simulink model "Current_torque_111"  (R2017b)
settings: Solver=ode45  StartTime=0.0  StopTime=3  MaxStep=1e-4  RelTol=1e-3  EnableMultiTasking=on
libraries: neural x38, fuzblock x6, simulink x1
(part 1 of 3)
settings Model: Creator=Tianfu Sun  LastModifiedBy=dachuan
settings DataIOCC: LimitDataPoints=on  SaveFormat=Array  SignalLoggingSaveFormat=ModelDataLogs
settings OptimizationCC: ExpressionDepthLimit=2147483647  LifeSpan=inf
settings DebuggingCC: UnderspecifiedInitializationDetection=Classic  MergeDetectMultiDrivingBlocksExec=none  SolverPrmCheckMsg=warning  FcnCallInpInsideContextMsg=warning  StateNameClashWarn=warning  StrictBusMsg=Warning  SFUnexpectedBacktrackingDiag=warning  SFNoUnconditionalDefaultTransitionDiag=warning  SFExecutionAtInitializationDiag=none
settings HardwareCC: ProdBitPerPointer=32  ProdBitPerSizeT=32  ProdBitPerPtrDiffT=32  ProdLargestAtomicFloat=None  ProdIntDivRoundTo=Undefined  ProdEndianess=Unspecified  ProdWordSize=32  ProdHWDeviceType=32-bit Generic
settings ModelReferenceCC: PropagateSignalLabelsOutOfModel=off
settings SFSimCC: SimParseCustomCode=off
settings CodeAppCC: StateflowObjectComments=on
settings GRTTargetCC: TargetLangStandard=C89/C90 (ANSI)  GeneratePreprocessorConditionals=Disable all  CombineOutputUpdateFcns=off  GRTInterface=on
settings ConfigComp: CovMetricSettings=dw  CovHtmlReporting=on  CovSaveCumulativeToWorkspaceVar=on  CovSaveSingleToWorkspaceVar=on  CovExternalEMLEnable=off

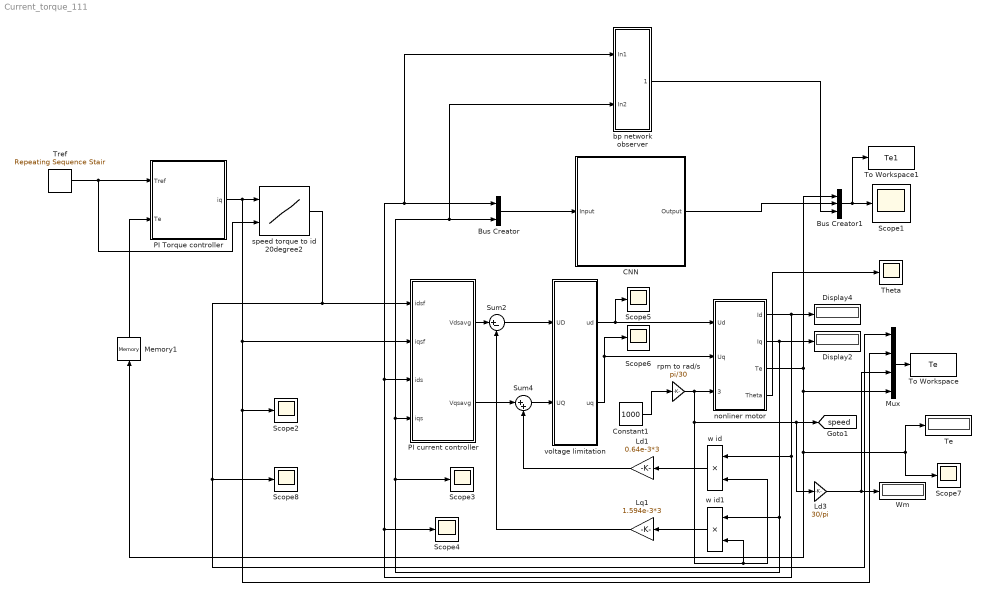
== system Current_torque_111 ==
  Bus Creator : BusCreator  Inputs=2
  Bus Creator1 : BusCreator  Inputs=3
  CNN : Subsystem
      mask help: Custom Neural Network
      mask Display: e = 0.06;c1 = [120 150 230]/255;c2 = ([120 150 230]+0)/383;c3 = ([120 150 230]+128)/383;patch([0 1 1 0],[0 0 1 1],c1);patch([0 1 1 1-e 1-e 0+e],[0 0 1 1-e 0+e 0+e],c2);patch([0 0 1 1-e 0+e 0+e],[0 1 1 1-e 1-e 0+e],c3);plot([0 1 1 0 0],[0 0 1 1 0]);fprintf('NNET');port_label('input',1,' Input');port_label('output',1,'Output ');
  Constant1 : Constant  Value=1000
  Display2 : Display
  Display4 : Display
  Ld1 : Gain  Gain=0.64e-3*3
  Ld3 : Gain  Gain=30/pi
  Lq1 : Gain  Gain=1.594e-3*3
  Memory1 : Memory  InheritSampleTime=on  LinearizeMemory=on  LinearizeAsDelay=on
  Mux : Mux
  PI Torque controller : Subsystem  mask{Kp=0.01, Ki=300}
  PI current controller : Subsystem  mask{Kp=2*1, Ki=40*1}
  Scope{1..8} (8 alike) : Scope
      Scope1 mask Display: e = 0.06;c1 = [120 230 180]/255;c2 = ([120 230 180]+0)/(256+128);c3 = ([120 230 180]+128)/(256+128);patch([0 1 1 0],[0 0 1 1],c1);patch([0 1 1 1-e 1-e 0+e],[0 0 1 1-e 0+e 0+e],c2);patch([0 0 1 1-e 0+e 0+e],[0 1 1 1-e 1-e 0+e],c3);plot([0 1 1 0 0],[0 0 1 1 0]);plot([0.15 0.85 0.85 0.15 0.15],[0.5 0.5 0.85 0.85 0.5]);
  Sum2 : Sum  Inputs=|+-
  Sum4 : Sum  Inputs=|++
  Te : Display
  Theta : Scope
  To Workspace : ToWorkspace  VariableName=Te  SaveFormat=Structure With Time  SampleTime=-1
  To Workspace1 : ToWorkspace  VariableName=Te1  SaveFormat=Structure With Time  SampleTime=-1
  Tref : simulink/Sources/Repeating Sequence Stair  OutValues=[10,20,30]  tsamp=1  OutMin=[]  OutMax=[]  OutDataTypeStr=double  OutputDataTypeScalingMode=double  OutDataType=fixdt(0,8)  ConRadixGroup=Best Precision: Vector-wise  OutScaling=2^-12
  Wm : Display
  "bp network observer " : Subsystem
  "nonliner motor " : Subsystem
  rpm to rad/s : Gain  Gain=pi/30
  speed torque to id 20degree2 : Lookup2D  RowIndex=[0,1,2,3,4,5,6,7,8,9,10,11,12,13,14,15,16,17,18,19,20,21,22,23,24,25,26,27,28,29,30,31,32,33,34,35,36,37,38,39,40,41,42,43,44,45,46,47,48,49,50,51,52,53,54,55,56,57,58,59,60,61,62,63,64,65,66,67,68,69,70]  ColumnIndex=[0,100,200,300,400,500,600,700,800,900,1000,1100,1200,1300,1400,1500,1600,1700,1800,1900,2000,2100,2200,2300,2400,2500,2600,2700,2800,2900,3000,3100,3200,3300,3400,3500,3600,3700,3800,3900,4000,4100,4200,4300,4400,4500]  Table=[0.00,0.00,0.00,0.00,0.00,0.00,0.00,0.00,0.00,0.00,0.00,0.00,0.00,0.00,0.00,0.00,0.00,0.00,-6.04,-15.13,-22.66,-28.59,-34.00,-38.97,-43.38,-47.39,-51.09,-54.51,-57.70,-60.67,-63.45,-66.06,-68.52,-70.82,-72.98,-75.03,-76.96,-78.79,-80.53,-82.19,-83.77,-85.27,-86.70,-88.07,-89.37,-90.62;-0.04,-0.04,-0.04,-0.04,-0.04,-0.04,-0.04,-0.04,-0.04,-0.04,-0.04,-0.04,-0.04,-0.04,-0.04,-0.04,-0.04,-0.04,-6.26,-15.35,-22.84,-28.77,-34.20,-39.17,-43.56,-47.58,-51.29,-54.71,-57.90,-60.85,-63.69,-66.27,-68.72,-71.03,-73.20,-75.24,-77.17,-79.00,-80.75,-82.41,-83.99,-85.49,-86.93,-88.29,-89.60,-90.85;-0.17,-0.17,-0.17,-0.17,-0.17,-0.17,-0.17,-0.17,-0.17,-0.17,-0.17,-0.17,-0.17,-0.17,-0.17,-0.17,-0.17,-0.17,-6.50,-15.61,-23.08,-29.00,-34.44,-39.41,-43.82,-47.82,-51.52,-54.96,-58.15,-61.12,-63.90,-66.53,-68.98,-71.28,-73.45,-75.49,-77.43,-79.26,-81.01,-82.67,-84.25,-85.76,-87.19,-88.56,-89.86,-91.11;-0.38,-0.38,-0.38,-0.38,-0.38,-0.38,-0.38,-0.38,-0.38,-0.38,-0.38,-0.38,-0.38,-0.38,-0.38,-0.38,-0.38,-0.38,-6.85,-15.98,-23.39,-29.31,-34.77,-39.74,-44.14,-48.15,-51.85,-55.28,-58.47,-61.45,-64.25,-66.85,-69.31,-71.61,-73.78,-75.83,-77.76,-79.60,-81.35,-83.01,-84.60,-86.10,-87.54,-88.91,-90.22,-91.47;-0.67,-0.67,-0.67,-0.67,-0.67,-0.67,-0.67,-0.67,-0.67,-0.67,-0.67,-0.67,-0.67,-0.67,-0.67,-0.67,-0.67,-0.67,-7.26,-16.42,-23.77,-29.70,-35.19,-40.14,-44.54,-48.54,-52.25,-55.69,-58.88,-61.86,-64.65,-67.27,-69.72,-72.03,-74.20,-76.25,-78.26,-80.03,-81.77,-83.45,-85.03,-86.53,-87.98,-89.35,-90.66,-91.92;-1.04,-1.04,-1.04,-1.04,-1.04,-1.04,-1.04,-1.04,-1.04,-1.04,-1.04,-1.04,-1.04,-1.04,-1.04,-1.04,-1.04,-1.04,-7.80,-16.98,-24.24,-30.17,-35.69,-40.64,-45.01,-49.03,-52.73,-56.17,-59.36,-62.35,-65.14,-67.76,-70.22,-72.52,-74.69,-76.75,-78.69,-80.54,-82.29,-83.96,-85.55,-87.06,-88.51,-89.88,-91.20,-92.44;-1.47,-1.47,-1.47,-1.47,-1.47,-1.47,-1.47,-1.47,-1.47,-1.47,-1.47,-1.47,-1.47,-1.47,-1.47,-1.47,-1.47,-1.47,-8.50,-17.64,-24.81,-30.73,-36.28,-41.21,-45.57,-49.59,-53.29,-56.74,-59.94,-62.91,-65.73,-68.33,-70.78,-73.09,-75.26,-77.33,-79.28,-81.13,-82.89,-84.56,-86.16,-87.67,-89.12,-90.50,-91.81,-93.07;-1.97,-1.97,-1.97,-1.97,-1.97,-1.97,-1.97,-1.97,-1.97,-1.97,-1.97,-1.97,-1.97,-1.97,-1.97,-1.97,-1.97,-1.97,-9.34,-18.44,-25.46,-31.42,-36.97,-41.86,-46.23,-50.23,-53.94,-57.38,-60.58,-63.57,-66.36,-68.98,-71.44,-73.75,-75.92,-77.99,-79.94,-81.80,-83.55,-85.23,-86.83,-88.35,-89.81,-91.20,-92.53,-93.79;-2.53,-2.53,-2.53,-2.53,-2.53,-2.53,-2.53,-2.53,-2.53,-2.53,-2.53,-2.53,-2.53,-2.53,-2.53,-2.53,-2.53,-2.53,-10.41,-19.38,-26.24,-32.22,-37.76,-42.61,-46.95,-50.96,-54.67,-58.11,-61.31,-64.29,-67.09,-69.70,-72.16,-74.47,-76.66,-78.73,-80.69,-82.55,-84.32,-86.01,-87.61,-89.14,-90.60,-91.99,-93.32,-94.59;-3.17,-3.17,-3.17,-3.17,-3.17,-3.17,-3.17,-3.17,-3.17,-3.17,-3.17,-3.17,-3.17,-3.17,-3.17,-3.17,-3.17,-3.17,-11.70,-20.49,-27.16,-33.16,-38.66,-43.45,-47.78,-51.78,-55.48,-58.92,-62.12,-65.10,-67.89,-70.51,-72.97,-75.29,-77.48,-79.55,-81.52,-83.39,-85.16,-86.85,-88.46,-90.00,-91.46,-92.86,-94.20,-95.49;-3.83,-3.83,-3.83,-3.83,-3.83,-3.83,-3.83,-3.83,-3.83,-3.83,-3.83,-3.83,-3.83,-3.83,-3.83,-3.83,-3.83,-3.83,-13.18,-21.74,-28.24,-34.24,-39.67,-44.40,-48.70,-52.69,-56.38,-59.82,-63.01,-65.99,-68.77,-71.39,-73.85,-76.17,-78.37,-80.46,-82.43,-84.31,-86.09,-87.78,-89.40,-90.94,-92.41,-93.82,-95.17,-96.47;-4.53,-4.53,-4.53,-4.53,-4.53,-4.53,-4.53,-4.53,-4.53,-4.53,-4.53,-4.53,-4.53,-4.53,-4.53,-4.53,-4.53,-3.55,-14.78,-23.08,-29.48,-35.47,-40.79,-45.45,-49.73,-53.70,-57.38,-60.80,-63.99,-66.96,-69.74,-72.36,-74.82,-77.15,-79.35,-81.44,-83.42,-85.30,-87.09,-88.80,-90.42,-91.98,-93.46,-94.88,-96.24,-97.54;-5.30,-5.30,-5.30,-5.30,-5.30,-5.30,-5.30,-5.30,-5.30,-5.30,-5.30,-5.30,-5.30,-5.30,-5.30,-5.30,-5.30,-5.14,-16.37,-24.42,-30.82,-36.80,-42.00,-46.61,-50.86,-54.82,-58.48,-61.89,-65.06,-68.02,-70.80,-73.41,-75.88,-78.21,-80.42,-82.51,-84.50,-86.39,-88.19,-89.90,-91.53,-93.09,-94.59,-96.02,-97.39,-98.71;-6.12,-6.12,-6.12,-6.12,-6.12,-6.12,-6.12,-6.12,-6.12,-6.12,-6.12,-6.12 ...(+19641 chars)]
  voltage limitation : Subsystem  mask{Umax=120/sqrt(3)}
  w id : Product  RndMeth=Zero
  w id1 : Product  RndMeth=Zero
  tag scope: speed=global
  wires:
  PI current controller/1("Vdsavg ") -> Sum2/1
  PI current controller/2(Vqsavg) -> Sum4/1
  voltage limitation/1(ud) -> Scope5/1, "nonliner motor "/1(Ud)
  voltage limitation/2(uq) -> Scope6/1, "nonliner motor "/2(Uq)
  Sum2/1 -> voltage limitation/1(UD)
  Sum4/1 -> voltage limitation/2(UQ)
  w id/1 -> Ld1/1
  w id1/1 -> Lq1/1
  Ld1/1 -> Sum4/2
  Lq1/1 -> Sum2/2
  rpm to rad/s/1 -> w id1/2, w id/2, [speed], Ld3/1, "nonliner motor "/3(Wm_in)
  Ld3/1 -> Mux/3, Wm/1
  Constant1/1 -> rpm to rad/s/1
  speed torque to id 20degree2/1 -> Scope8/1, Mux/1, PI current controller/1(idsf)
  Bus Creator1/1 -> Scope1/1, To Workspace1/1
  Mux/1 -> To Workspace/1
  "nonliner motor "/3(Te) -> Bus Creator1/1, Mux/4, Memory1/1, Te/1, Scope7/1
  Bus Creator/1 -> CNN/1(Input)
  "nonliner motor "/4(Theta) -> Theta/1
  "nonliner motor "/2(Iq) -> Display2/1, "bp network observer "/2(In2), Bus Creator/2, PI current controller/4(iqs), Scope3/1, w id1/1
  Tref/1 -> PI Torque controller/1(Tref), speed torque to id 20degree2/2
  CNN/1(Output) -> Bus Creator1/2
  PI Torque controller/1("iq ") -> speed torque to id 20degree2/1, Scope2/1, Mux/2, PI current controller/2(iqsf)
  Memory1/1 -> PI Torque controller/2(Te)
  "nonliner motor "/1(Id) -> Scope4/1, "bp network observer "/1(In1), Bus Creator/1, PI current controller/3(ids), w id/1, Display4/1
  "bp network observer "/1(Out1) -> Bus Creator1/3

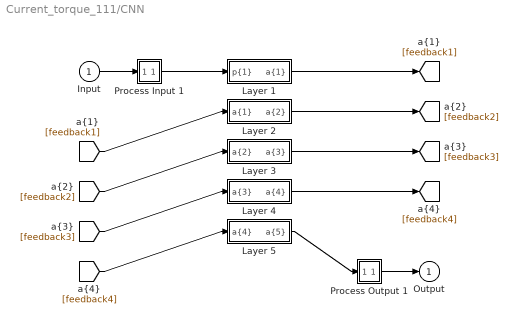
== system Current_torque_111/CNN ==
  Input : Inport  PortDimensions=2
      mask Display: e = 0.06;c1 = [120 230 180]/255;c2 = ([120 230 180]+0)/(256+128);c3 = ([120 230 180]+128)/(256+128);patch([0 1 1 0],[0 0 1 1],c1);patch([0 1 1 1-e 1-e 0+e],[0 0 1 1-e 0+e 0+e],c2);patch([0 0 1 1-e 0+e 0+e],[0 1 1 1-e 1-e 0+e],c3);plot([0 1 1 0 0],[0 0 1 1 0]);
  Layer 1 : Subsystem
      mask Display: e = 0.06;c1 = [120 150 230]/255;c2 = ([120 150 230]+0)/383;c3 = ([120 150 230]+128)/383;patch([0 1 1 0],[0 0 1 1],c1);patch([0 1 1 1-e 1-e 0+e],[0 0 1 1-e 0+e 0+e],c2);patch([0 0 1 1-e 0+e 0+e],[0 1 1 1-e 1-e 0+e],c3);plot([0 1 1 0 0],[0 0 1 1 0]);
  Layer 2 : Subsystem
      mask Display: e = 0.06;c1 = [120 150 230]/255;c2 = ([120 150 230]+0)/383;c3 = ([120 150 230]+128)/383;patch([0 1 1 0],[0 0 1 1],c1);patch([0 1 1 1-e 1-e 0+e],[0 0 1 1-e 0+e 0+e],c2);patch([0 0 1 1-e 0+e 0+e],[0 1 1 1-e 1-e 0+e],c3);plot([0 1 1 0 0],[0 0 1 1 0]);
  Layer 3 : Subsystem
      mask Display: e = 0.06;c1 = [120 150 230]/255;c2 = ([120 150 230]+0)/383;c3 = ([120 150 230]+128)/383;patch([0 1 1 0],[0 0 1 1],c1);patch([0 1 1 1-e 1-e 0+e],[0 0 1 1-e 0+e 0+e],c2);patch([0 0 1 1-e 0+e 0+e],[0 1 1 1-e 1-e 0+e],c3);plot([0 1 1 0 0],[0 0 1 1 0]);
  Layer 4 : Subsystem
      mask Display: e = 0.06;c1 = [120 150 230]/255;c2 = ([120 150 230]+0)/383;c3 = ([120 150 230]+128)/383;patch([0 1 1 0],[0 0 1 1],c1);patch([0 1 1 1-e 1-e 0+e],[0 0 1 1-e 0+e 0+e],c2);patch([0 0 1 1-e 0+e 0+e],[0 1 1 1-e 1-e 0+e],c3);plot([0 1 1 0 0],[0 0 1 1 0]);
  Layer 5 : Subsystem
      mask Display: e = 0.06;c1 = [120 150 230]/255;c2 = ([120 150 230]+0)/383;c3 = ([120 150 230]+128)/383;patch([0 1 1 0],[0 0 1 1],c1);patch([0 1 1 1-e 1-e 0+e],[0 0 1 1-e 0+e 0+e],c2);patch([0 0 1 1-e 0+e 0+e],[0 1 1 1-e 1-e 0+e],c3);plot([0 1 1 0 0],[0 0 1 1 0]);
  Process Input 1 : Subsystem
      mask Display: e = 0.06;c1 = [120 150 230]/255;c2 = ([120 150 230]+0)/383;c3 = ([120 150 230]+128)/383;patch([0 1 1 0],[0 0 1 1],c1);patch([0 1 1 1-e 1-e 0+e],[0 0 1 1-e 0+e 0+e],c2);patch([0 0 1 1-e 0+e 0+e],[0 1 1 1-e 1-e 0+e],c3);plot([0 1 1 0 0],[0 0 1 1 0]);
  Process Output 1 : Subsystem
      mask Display: e = 0.06;c1 = [120 150 230]/255;c2 = ([120 150 230]+0)/383;c3 = ([120 150 230]+128)/383;patch([0 1 1 0],[0 0 1 1],c1);patch([0 1 1 1-e 1-e 0+e],[0 0 1 1-e 0+e 0+e],c2);patch([0 0 1 1-e 0+e 0+e],[0 1 1 1-e 1-e 0+e],c3);plot([0 1 1 0 0],[0 0 1 1 0]);
  Output : Outport  InitialOutput=0
      mask Display: e = 0.06;c1 = [120 230 180]/255;c2 = ([120 230 180]+0)/(256+128);c3 = ([120 230 180]+128)/(256+128);patch([0 1 1 0],[0 0 1 1],c1);patch([0 1 1 1-e 1-e 0+e],[0 0 1 1-e 0+e 0+e],c2);patch([0 0 1 1-e 0+e 0+e],[0 1 1 1-e 1-e 0+e],c3);plot([0 1 1 0 0],[0 0 1 1 0]);
  wires:
  Layer 5/1("a{5}") -> Process Output 1/1(a)
  [feedback4] -> Layer 5/1("a{4} ")
  Layer 4/1("a{4}") -> [feedback4]
  [feedback3] -> Layer 4/1("a{3} ")
  Layer 3/1("a{3}") -> [feedback3]
  [feedback2] -> Layer 3/1("a{2} ")
  Layer 2/1("a{2}") -> [feedback2]
  [feedback1] -> Layer 2/1("a{1} ")
  Layer 1/1("a{1}") -> [feedback1]
  Process Input 1/1(p) -> Layer 1/1("p{1}")
  Process Output 1/1(y) -> Output/1
  Input/1 -> Process Input 1/1(x)

== system Current_torque_111/PI Torque controller ==
  Tref : Inport
  Te : Inport  Port=2
  PI-Te-iq : Subsystem
  Sum : Sum  Inputs=|+-
  TE : Scope
  iq : Scope
  "iq " : Outport
  wires:
  Tref/1 -> Sum/1
  Te/1 -> Sum/2
  Sum/1 -> TE/1, PI-Te-iq/1(In1)
  PI-Te-iq/1(iq) -> iq/1, "iq "/1

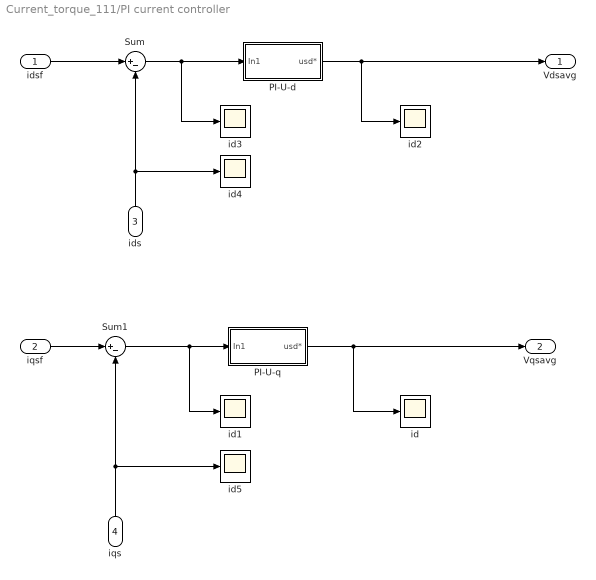
== system Current_torque_111/PI current controller ==
  idsf : Inport
  iqsf : Inport  Port=2
  ids : Inport  Port=3
  iqs : Inport  Port=4
  PI-U-d : Subsystem
  PI-U-q : Subsystem
  Sum : Sum  Inputs=|+-
  Sum1 : Sum  Inputs=|+-
  id{,1..5} (6 alike) : Scope
  "Vdsavg " : Outport
  Vqsavg : Outport  Port=2
  wires:
  PI-U-q/1(usd*) -> Vqsavg/1, id/1
  PI-U-d/1(usd*) -> "Vdsavg "/1, id2/1
  iqsf/1 -> Sum1/1
  Sum1/1 -> PI-U-q/1(In1), id1/1
  iqs/1 -> Sum1/2, id5/1
  Sum/1 -> PI-U-d/1(In1), id3/1
  ids/1 -> Sum/2, id4/1
  idsf/1 -> Sum/1

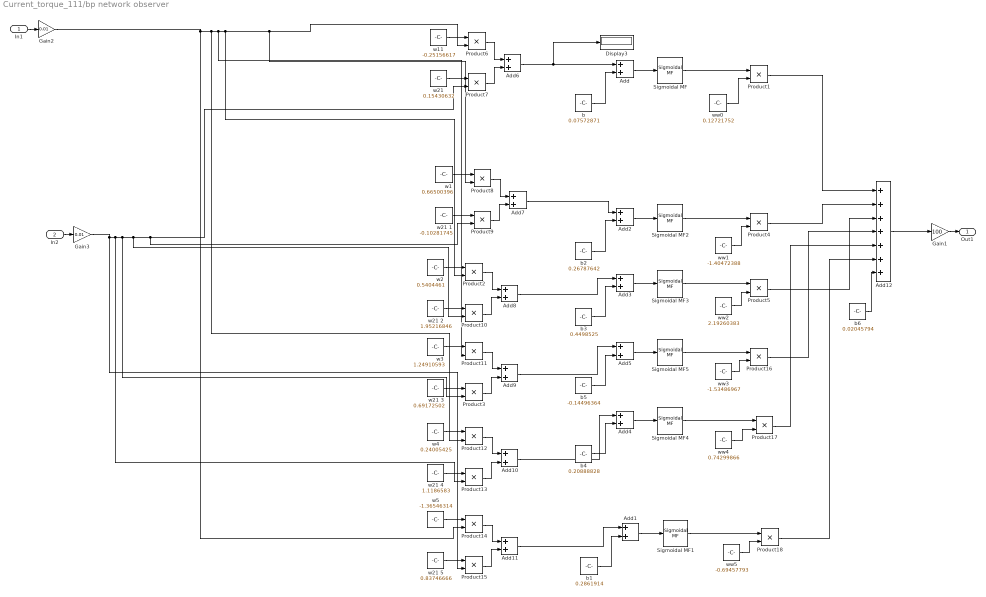
== system Current_torque_111/bp network observer  ==
  In1 : Inport
  In2 : Inport  Port=2
  Add{,1..11} (12 alike) : Sum
  Add12 : Sum  Inputs=+++++++
  Display3 : Display
  Gain1 : Gain  Gain=100
  Gain2 : Gain  Gain=0.01
  Gain3 : Gain  Gain=0.01
  Product{1..18} (18 alike) : Product
  Sigmoidal MF{,1..5} (6 alike) : fuzblock/Membership  Functions/Sigmoidal MF  a=1  c=0
      settings: SourceProductName=Fuzzy Logic Toolbox  SourceProductBaseCode=FL
  b : Constant  Value=0.07572871
  b1 : Constant  Value=0.2861914
  b2 : Constant  Value=0.26787642
  b3 : Constant  Value=0.4498525
  b4 : Constant  Value=0.20888828
  b5 : Constant  Value=-0.14496364
  b6 : Constant  Value=0.02045794
  w1 : Constant  Value=0.66500396
  w11 : Constant  Value=-0.25156617
  w2 : Constant  Value=0.5404461
  "w21 " : Constant  Value=0.15430632
  w21 1 : Constant  Value=-0.10281745
  w21 2 : Constant  Value=1.95216846
  w21 3 : Constant  Value=0.69172502
  w21 4 : Constant  Value=1.1186583
  w21 5 : Constant  Value=0.83746666
  w3 : Constant  Value=1.24910593
  w4 : Constant  Value=0.24005425
  w5 : Constant  Value=-1.36546314
  ww0 : Constant  Value=0.12721752
  ww1 : Constant  Value=-1.40472388
  ww2 : Constant  Value=2.19260383
  ww3 : Constant  Value=-1.53486967
  ww4 : Constant  Value=0.74299866
  ww5 : Constant  Value=-0.69457793
  Out1 : Outport
  wires:
  Add2/1 -> Sigmoidal MF2/1
  Add12/1 -> Gain1/1
  Sigmoidal MF1/1 -> Product18/1
  Gain2/1 -> Product14/2, Product12/2, Product11/2, Product2/2, Product8/2, Product6/2
  ww0/1 -> Product1/2
  Product5/1 -> Add12/3
  ww2/1 -> Product5/2
  Add10/1 -> Add4/1
  b2/1 -> Add2/2
  Product16/1 -> Add12/4
  Sigmoidal MF4/1 -> Product17/1
  ww5/1 -> Product18/2
  Gain3/1 -> Product15/2, Product13/2, Product3/2, Product10/2, Product9/2, Product7/2
  b4/1 -> Add4/2
  Product6/1 -> Add6/1
  Add6/1 -> Display3/1, Add/1
  Add7/1 -> Add2/1
  w3/1 -> Product11/1
  ww3/1 -> Product16/2
  Sigmoidal MF3/1 -> Product5/1
  Add4/1 -> Sigmoidal MF4/1
  Product8/1 -> Add7/1
  w2/1 -> Product2/1
  Product11/1 -> Add9/1
  w21 3/1 -> Product3/1
  b6/1 -> Add12/7
  Product18/1 -> Add12/6
  Add8/1 -> Add3/1
  ww1/1 -> Product4/2
  Add5/1 -> Sigmoidal MF5/1
  w21 2/1 -> Product10/1
  Product10/1 -> Add8/2
  Product3/1 -> Add9/2
  w21 1/1 -> Product9/1
  Sigmoidal MF/1 -> Product1/1
  "w21 "/1 -> Product7/1
  Product2/1 -> Add8/1
  ww4/1 -> Product17/2
  b/1 -> Add/2
  Product9/1 -> Add7/2
  Add3/1 -> Sigmoidal MF3/1
  Sigmoidal MF5/1 -> Product16/1
  w1/1 -> Product8/1
  Product15/1 -> Add11/2
  Add9/1 -> Add5/1
  Product17/1 -> Add12/5
  w21 4/1 -> Product13/1
  Product12/1 -> Add10/1
  Add/1 -> Sigmoidal MF/1
  Product7/1 -> Add6/2
  b3/1 -> Add3/2
  Product13/1 -> Add10/2
  w5/1 -> Product14/1
  Product4/1 -> Add12/2
  w21 5/1 -> Product15/1
  Add1/1 -> Sigmoidal MF1/1
  Product1/1 -> Add12/1
  b5/1 -> Add5/2
  b1/1 -> Add1/2
  Sigmoidal MF2/1 -> Product4/1
  w11/1 -> Product6/1
  w4/1 -> Product12/1
  Add11/1 -> Add1/1
  Product14/1 -> Add11/1
  In2/1 -> Gain3/1
  In1/1 -> Gain2/1
  Gain1/1 -> Out1/1

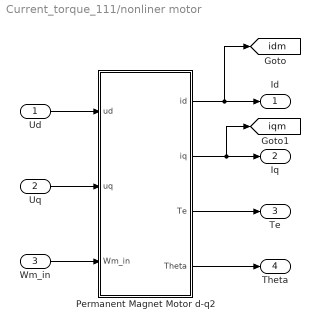
== system Current_torque_111/nonliner motor  ==
  Ud : Inport
  Uq : Inport  Port=2
  Wm_in : Inport  Port=3
  Permanent Magnet Motor d-q2 : Subsystem  mask{Rs=0.0512, P=3, J=0.0073, F=0}
      mask prompts: Rs "Stator Resistance (Ohm)"; P "Pole Pairs"; J "Inertia Torque"; F "Friction"
  Id : Outport
  Iq : Outport  Port=2
  Te : Outport  Port=3
  Theta : Outport  Port=4
  tag scope: idm=global, iqm=global
  wires:
  Permanent Magnet Motor d-q2/3(Te) -> Te/1
  Permanent Magnet Motor d-q2/2(iq) -> [iqm], Iq/1
  Permanent Magnet Motor d-q2/1(id) -> [idm], Id/1
  Wm_in/1 -> Permanent Magnet Motor d-q2/3(Wm_in)
  Uq/1 -> Permanent Magnet Motor d-q2/2(uq)
  Ud/1 -> Permanent Magnet Motor d-q2/1(ud)
  Permanent Magnet Motor d-q2/4(Theta) -> Theta/1

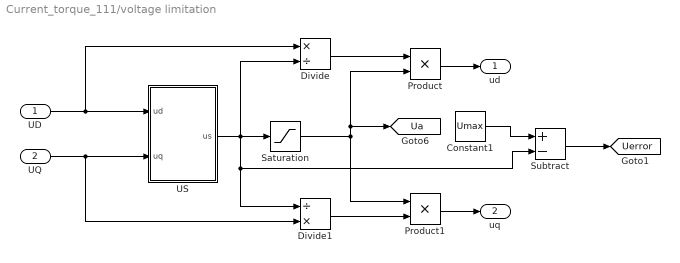
== system Current_torque_111/voltage limitation ==
  UD : Inport
  UQ : Inport  Port=2
  Constant1 : Constant  Value=Umax
  Divide : Product  Inputs=*/
  Divide1 : Product  Inputs=/*
  Product : Product  RndMeth=Zero
  Product1 : Product  RndMeth=Zero
  Saturation : Saturate  UpperLimit=Umax  LowerLimit=0
  Subtract : Sum  Inputs=+-
  US : MATLAB Function  TreatAsAtomicUnit=on
  ud : Outport
  uq : Outport  Port=2
  tag scope: Ua=global, Uerror=global
  wires:
  Product1/1 -> uq/1
  Divide1/1 -> Product1/2
  Divide/1 -> Product/1
  Product/1 -> ud/1
  US/1(us) -> Subtract/2, Divide1/1, Divide/2, Saturation/1
  UD/1 -> Divide/1, US/1(ud)
  UQ/1 -> Divide1/2, US/2(uq)
  Constant1/1 -> Subtract/1
  Saturation/1 -> Product1/1, [Ua], Product/2
  Subtract/1 -> [Uerror]

== system Current_torque_111/CNN/Layer 1 ==
  "p{1}" : Inport  PortDimensions=2
      mask Display: e = 0.06;c1 = [120 230 180]/255;c2 = ([120 230 180]+0)/(256+128);c3 = ([120 230 180]+128)/(256+128);patch([0 1 1 0],[0 0 1 1],c1);patch([0 1 1 1-e 1-e 0+e],[0 0 1 1-e 0+e 0+e],c2);patch([0 0 1 1-e 0+e 0+e],[0 1 1 1-e 1-e 0+e],c3);plot([0 1 1 0 0],[0 0 1 1 0]);
  Delays 1 : Subsystem
      mask Display: e = 0.06;c1 = [120 150 230]/255;c2 = ([120 150 230]+0)/383;c3 = ([120 150 230]+128)/383;patch([0 1 1 0],[0 0 1 1],c1);patch([0 1 1 1-e 1-e 0+e],[0 0 1 1-e 0+e 0+e],c2);patch([0 0 1 1-e 0+e 0+e],[0 1 1 1-e 1-e 0+e],c3);plot([0 1 1 0 0],[0 0 1 1 0]);disp('0');
  "IW{1,1}" : Subsystem
      mask Display: e = 0.06;c1 = [120 150 230]/255;c2 = ([120 150 230]+0)/383;c3 = ([120 150 230]+128)/383;patch([0 1 1 0],[0 0 1 1],c1);patch([0 1 1 1-e 1-e 0+e],[0 0 1 1-e 0+e 0+e],c2);patch([0 0 1 1-e 0+e 0+e],[0 1 1 1-e 1-e 0+e],c3);plot([0 1 1 0 0],[0 0 1 1 0]);disp('W');
  "b{1}" : Constant  Value=[-3.239525138320037189743061389890499413013458251953125;-2.918799402758903926979883181047625839710235595703125;1.812716926213318924254735975409857928752899169921875;-1.01904056907273687926362981670536100864410400390625;-1.3780316727236776586096311802975833415985107421875;0.430711173271133562767687408268102444708347320556640625;-0.3296334238442766295662522679776884615421295166015625;-0.03799616971614404314916413341052248142659664154052734375;0.618674101925375197197354282252490520477294921875;1.9290423818612811857065025833435356616973876953125]
      mask Display: e = 0.06;c1 = [120 150 230]/255;c2 = ([120 150 230]+0)/383;c3 = ([120 150 230]+128)/383;patch([0 1 1 0],[0 0 1 1],c1);patch([0 1 1 1-e 1-e 0+e],[0 0 1 1-e 0+e 0+e],c2);patch([0 0 1 1-e 0+e 0+e],[0 1 1 1-e 1-e 0+e],c3);plot([0 1 1 0 0],[0 0 1 1 0]);disp('b');
  netsum : Sum  Inputs=2  SaturateOnIntegerOverflow=on  InputSameDT=on  OutDataTypeStr=Inherit: Same as first input
      mask Display: e = 0.06;c1 = [120 150 230]/255;c2 = ([120 150 230]+0)/383;c3 = ([120 150 230]+128)/383;patch([0 1 1 0],[0 0 1 1],c1);patch([0 1 1 1-e 1-e 0+e],[0 0 1 1-e 0+e 0+e],c2);patch([0 0 1 1-e 0+e 0+e],[0 1 1 1-e 1-e 0+e],c3);plot([0 1 1 0 0],[0 0 1 1 0]);disp('+');
  tansig : neural/Transfer Functions/tansig
  "a{1}" : Outport  InitialOutput=[0;0;0;0;0;0;0;0;0;0]
      mask Display: e = 0.06;c1 = [120 230 180]/255;c2 = ([120 230 180]+0)/(256+128);c3 = ([120 230 180]+128)/(256+128);patch([0 1 1 0],[0 0 1 1],c1);patch([0 1 1 1-e 1-e 0+e],[0 0 1 1-e 0+e 0+e],c2);patch([0 0 1 1-e 0+e 0+e],[0 1 1 1-e 1-e 0+e],c3);plot([0 1 1 0 0],[0 0 1 1 0]);
  wires:
  tansig/1 -> "a{1}"/1
  netsum/1 -> tansig/1
  "b{1}"/1 -> netsum/2
  "IW{1,1}"/1("iz{1,1}") -> netsum/1
  Delays 1/1("pd{1,1}") -> "IW{1,1}"/1("pd{1,1}")
  "p{1}"/1 -> Delays 1/1("p{1}")

== system Current_torque_111/CNN/Layer 2 ==
  "a{1} " : Inport  PortDimensions=10
      mask Display: e = 0.06;c1 = [120 230 180]/255;c2 = ([120 230 180]+0)/(256+128);c3 = ([120 230 180]+128)/(256+128);patch([0 1 1 0],[0 0 1 1],c1);patch([0 1 1 1-e 1-e 0+e],[0 0 1 1-e 0+e 0+e],c2);patch([0 0 1 1-e 0+e 0+e],[0 1 1 1-e 1-e 0+e],c3);plot([0 1 1 0 0],[0 0 1 1 0]);
  Delays 1 : Subsystem
      mask Display: e = 0.06;c1 = [120 150 230]/255;c2 = ([120 150 230]+0)/383;c3 = ([120 150 230]+128)/383;patch([0 1 1 0],[0 0 1 1],c1);patch([0 1 1 1-e 1-e 0+e],[0 0 1 1-e 0+e 0+e],c2);patch([0 0 1 1-e 0+e 0+e],[0 1 1 1-e 1-e 0+e],c3);plot([0 1 1 0 0],[0 0 1 1 0]);disp('0');
  "LW{2,1}" : Subsystem
      mask Display: e = 0.06;c1 = [120 150 230]/255;c2 = ([120 150 230]+0)/383;c3 = ([120 150 230]+128)/383;patch([0 1 1 0],[0 0 1 1],c1);patch([0 1 1 1-e 1-e 0+e],[0 0 1 1-e 0+e 0+e],c2);patch([0 0 1 1-e 0+e 0+e],[0 1 1 1-e 1-e 0+e],c3);plot([0 1 1 0 0],[0 0 1 1 0]);disp('W');
  "b{2}" : Constant  Value=[-1.24188173021034753418234686250798404216766357421875;0.7077197302398625655683872537338174879550933837890625;-1.817597398904509997663581089000217616558074951171875;1.8918644710342296111349469356355257332324981689453125;-1.272621624203331247571213680203072726726531982421875;-0.10767420339551490859886229145558900199830532073974609375;0.62462652909750004948108426106045953929424285888671875;0.466433564075144080351975617304560728371143341064453125;1.8725615616267574647935134635190479457378387451171875;-1.1378899311561376794799116396461613476276397705078125]
      mask Display: e = 0.06;c1 = [120 150 230]/255;c2 = ([120 150 230]+0)/383;c3 = ([120 150 230]+128)/383;patch([0 1 1 0],[0 0 1 1],c1);patch([0 1 1 1-e 1-e 0+e],[0 0 1 1-e 0+e 0+e],c2);patch([0 0 1 1-e 0+e 0+e],[0 1 1 1-e 1-e 0+e],c3);plot([0 1 1 0 0],[0 0 1 1 0]);disp('b');
  netsum : Sum  Inputs=2  SaturateOnIntegerOverflow=on  InputSameDT=on  OutDataTypeStr=Inherit: Same as first input
      mask Display: e = 0.06;c1 = [120 150 230]/255;c2 = ([120 150 230]+0)/383;c3 = ([120 150 230]+128)/383;patch([0 1 1 0],[0 0 1 1],c1);patch([0 1 1 1-e 1-e 0+e],[0 0 1 1-e 0+e 0+e],c2);patch([0 0 1 1-e 0+e 0+e],[0 1 1 1-e 1-e 0+e],c3);plot([0 1 1 0 0],[0 0 1 1 0]);disp('+');
  tansig : neural/Transfer Functions/tansig
  "a{2}" : Outport  InitialOutput=[0;0;0;0;0;0;0;0;0;0]
      mask Display: e = 0.06;c1 = [120 230 180]/255;c2 = ([120 230 180]+0)/(256+128);c3 = ([120 230 180]+128)/(256+128);patch([0 1 1 0],[0 0 1 1],c1);patch([0 1 1 1-e 1-e 0+e],[0 0 1 1-e 0+e 0+e],c2);patch([0 0 1 1-e 0+e 0+e],[0 1 1 1-e 1-e 0+e],c3);plot([0 1 1 0 0],[0 0 1 1 0]);
  wires:
  tansig/1 -> "a{2}"/1
  netsum/1 -> tansig/1
  "b{2}"/1 -> netsum/2
  "LW{2,1}"/1("lz{2,1}") -> netsum/1
  Delays 1/1("pd{2,1}") -> "LW{2,1}"/1("ad{2,1}")
  "a{1} "/1 -> Delays 1/1("p{2}")

== system Current_torque_111/CNN/Layer 3 ==
  "a{2} " : Inport  PortDimensions=10
      mask Display: e = 0.06;c1 = [120 230 180]/255;c2 = ([120 230 180]+0)/(256+128);c3 = ([120 230 180]+128)/(256+128);patch([0 1 1 0],[0 0 1 1],c1);patch([0 1 1 1-e 1-e 0+e],[0 0 1 1-e 0+e 0+e],c2);patch([0 0 1 1-e 0+e 0+e],[0 1 1 1-e 1-e 0+e],c3);plot([0 1 1 0 0],[0 0 1 1 0]);
  Delays 1 : Subsystem
      mask Display: e = 0.06;c1 = [120 150 230]/255;c2 = ([120 150 230]+0)/383;c3 = ([120 150 230]+128)/383;patch([0 1 1 0],[0 0 1 1],c1);patch([0 1 1 1-e 1-e 0+e],[0 0 1 1-e 0+e 0+e],c2);patch([0 0 1 1-e 0+e 0+e],[0 1 1 1-e 1-e 0+e],c3);plot([0 1 1 0 0],[0 0 1 1 0]);disp('0');
  "LW{3,2}" : Subsystem
      mask Display: e = 0.06;c1 = [120 150 230]/255;c2 = ([120 150 230]+0)/383;c3 = ([120 150 230]+128)/383;patch([0 1 1 0],[0 0 1 1],c1);patch([0 1 1 1-e 1-e 0+e],[0 0 1 1-e 0+e 0+e],c2);patch([0 0 1 1-e 0+e 0+e],[0 1 1 1-e 1-e 0+e],c3);plot([0 1 1 0 0],[0 0 1 1 0]);disp('W');
  "b{3}" : Constant  Value=[0.9180131550993786415659769772901199758052825927734375;1.2617393435598771578298737949808128178119659423828125;0.2738492960046488011727205957868136465549468994140625;0.72440653147026179414780244769644923508167266845703125;2.326106766171465611847679610946215689182281494140625]
      mask Display: e = 0.06;c1 = [120 150 230]/255;c2 = ([120 150 230]+0)/383;c3 = ([120 150 230]+128)/383;patch([0 1 1 0],[0 0 1 1],c1);patch([0 1 1 1-e 1-e 0+e],[0 0 1 1-e 0+e 0+e],c2);patch([0 0 1 1-e 0+e 0+e],[0 1 1 1-e 1-e 0+e],c3);plot([0 1 1 0 0],[0 0 1 1 0]);disp('b');
  netsum : Sum  Inputs=2  SaturateOnIntegerOverflow=on  InputSameDT=on  OutDataTypeStr=Inherit: Same as first input
      mask Display: e = 0.06;c1 = [120 150 230]/255;c2 = ([120 150 230]+0)/383;c3 = ([120 150 230]+128)/383;patch([0 1 1 0],[0 0 1 1],c1);patch([0 1 1 1-e 1-e 0+e],[0 0 1 1-e 0+e 0+e],c2);patch([0 0 1 1-e 0+e 0+e],[0 1 1 1-e 1-e 0+e],c3);plot([0 1 1 0 0],[0 0 1 1 0]);disp('+');
  tansig : neural/Transfer Functions/tansig
  "a{3}" : Outport  InitialOutput=[0;0;0;0;0]
      mask Display: e = 0.06;c1 = [120 230 180]/255;c2 = ([120 230 180]+0)/(256+128);c3 = ([120 230 180]+128)/(256+128);patch([0 1 1 0],[0 0 1 1],c1);patch([0 1 1 1-e 1-e 0+e],[0 0 1 1-e 0+e 0+e],c2);patch([0 0 1 1-e 0+e 0+e],[0 1 1 1-e 1-e 0+e],c3);plot([0 1 1 0 0],[0 0 1 1 0]);
  wires:
  tansig/1 -> "a{3}"/1
  netsum/1 -> tansig/1
  "b{3}"/1 -> netsum/2
  "LW{3,2}"/1("lz{3,2}") -> netsum/1
  Delays 1/1("pd{3,2}") -> "LW{3,2}"/1("ad{3,2}")
  "a{2} "/1 -> Delays 1/1("p{3}")

== system Current_torque_111/CNN/Layer 4 ==
  "a{3} " : Inport  PortDimensions=5
      mask Display: e = 0.06;c1 = [120 230 180]/255;c2 = ([120 230 180]+0)/(256+128);c3 = ([120 230 180]+128)/(256+128);patch([0 1 1 0],[0 0 1 1],c1);patch([0 1 1 1-e 1-e 0+e],[0 0 1 1-e 0+e 0+e],c2);patch([0 0 1 1-e 0+e 0+e],[0 1 1 1-e 1-e 0+e],c3);plot([0 1 1 0 0],[0 0 1 1 0]);
  Delays 1 : Subsystem
      mask Display: e = 0.06;c1 = [120 150 230]/255;c2 = ([120 150 230]+0)/383;c3 = ([120 150 230]+128)/383;patch([0 1 1 0],[0 0 1 1],c1);patch([0 1 1 1-e 1-e 0+e],[0 0 1 1-e 0+e 0+e],c2);patch([0 0 1 1-e 0+e 0+e],[0 1 1 1-e 1-e 0+e],c3);plot([0 1 1 0 0],[0 0 1 1 0]);disp('0');
  "LW{4,3}" : Subsystem
      mask Display: e = 0.06;c1 = [120 150 230]/255;c2 = ([120 150 230]+0)/383;c3 = ([120 150 230]+128)/383;patch([0 1 1 0],[0 0 1 1],c1);patch([0 1 1 1-e 1-e 0+e],[0 0 1 1-e 0+e 0+e],c2);patch([0 0 1 1-e 0+e 0+e],[0 1 1 1-e 1-e 0+e],c3);plot([0 1 1 0 0],[0 0 1 1 0]);disp('W');
  "b{4}" : Constant  Value=[0.1394331528539771436481231603465857915580272674560546875;1.2744858226537292278379709387081675231456756591796875;-0.5827314642944332323537537376978434622287750244140625;-2.33818016374659887191000962047837674617767333984375;-2.27611763547577350408346319454722106456756591796875]
      mask Display: e = 0.06;c1 = [120 150 230]/255;c2 = ([120 150 230]+0)/383;c3 = ([120 150 230]+128)/383;patch([0 1 1 0],[0 0 1 1],c1);patch([0 1 1 1-e 1-e 0+e],[0 0 1 1-e 0+e 0+e],c2);patch([0 0 1 1-e 0+e 0+e],[0 1 1 1-e 1-e 0+e],c3);plot([0 1 1 0 0],[0 0 1 1 0]);disp('b');
  netsum : Sum  Inputs=2  SaturateOnIntegerOverflow=on  InputSameDT=on  OutDataTypeStr=Inherit: Same as first input
      mask Display: e = 0.06;c1 = [120 150 230]/255;c2 = ([120 150 230]+0)/383;c3 = ([120 150 230]+128)/383;patch([0 1 1 0],[0 0 1 1],c1);patch([0 1 1 1-e 1-e 0+e],[0 0 1 1-e 0+e 0+e],c2);patch([0 0 1 1-e 0+e 0+e],[0 1 1 1-e 1-e 0+e],c3);plot([0 1 1 0 0],[0 0 1 1 0]);disp('+');
  tansig : neural/Transfer Functions/tansig
  "a{4}" : Outport  InitialOutput=[0;0;0;0;0]
      mask Display: e = 0.06;c1 = [120 230 180]/255;c2 = ([120 230 180]+0)/(256+128);c3 = ([120 230 180]+128)/(256+128);patch([0 1 1 0],[0 0 1 1],c1);patch([0 1 1 1-e 1-e 0+e],[0 0 1 1-e 0+e 0+e],c2);patch([0 0 1 1-e 0+e 0+e],[0 1 1 1-e 1-e 0+e],c3);plot([0 1 1 0 0],[0 0 1 1 0]);
  wires:
  tansig/1 -> "a{4}"/1
  netsum/1 -> tansig/1
  "b{4}"/1 -> netsum/2
  "LW{4,3}"/1("lz{4,3}") -> netsum/1
  Delays 1/1("pd{4,3}") -> "LW{4,3}"/1("ad{4,3}")
  "a{3} "/1 -> Delays 1/1("p{4}")
